simulink library "FasBtc"  (R2022b)
settings: Solver=VariableStepAuto  StartTime=0.0  StopTime=10.0  RelTol=1e-3
undefined symbols (not defined in the file or in its folder): Row
libraries: TuneVar x17, TOP x6, RTC x3, AudioStats x2, FeaturePath x2, HandyTextFile x2, dspmtrx3 x1
settings Model: Creator=kl13806  LastModifiedBy=kl13806
settings SolverCC: AlgebraicLoopSolver=TrustRegion
settings DebuggingCC: UnconnectedInputMsg=warning  UnconnectedOutputMsg=warning  UnconnectedLineMsg=warning  SFMachineParentedDataDiag=warning
settings ModelReferenceCC: EnableRefExpFcnMdlSchedulingChecks=on
settings RTWCC: DLArmComputeVersion=19.05

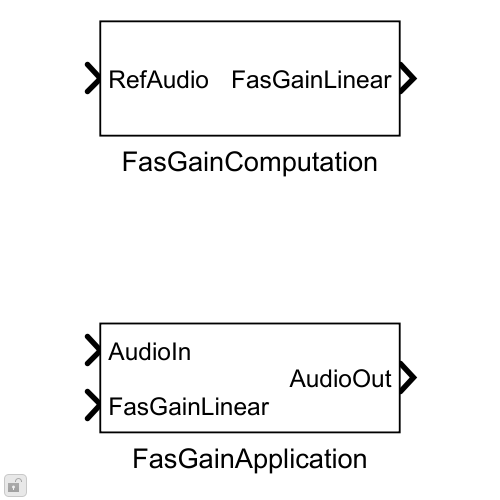
[thumbnail: Simulink's stored preview of the top-level diagram]
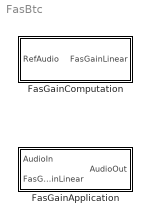
== system FasBtc ==
  FasGainApplication : Subsystem  mask(Blocklib FasGainApplication){Config=[], FeatureName=fas_application_}
      mask prompts: Config "FasGainApplicationConfig"; FeatureName "Feature path name:"
      mask help:
      | The Fresh Air Speaker (FAS) algorithm is designed to limit the output level of selected speaker channels. The level of the remaining channels remains unaffected. This has been implemented in 2 parts - a FAS gain computation block and a FAS gain application block. Refer to the Help section for more information.
      |
      | This limiting is only necessary when windows are open, leading to a reduction in the excursion range of the FAS transducers in order to prevent damage.
      mask init:
      | blkh=gcbh;
      | Config=BTConfig.Assert(blkh,Config);
      | Config.Validate();
      | BTConfig.InitSetFeatureIfPresent(blkh,'FeatureName');
      mask Help:
      | FAS Gain Application:
      | Description:
      | Applies the gain factor to the incoming audio after ramping it using a LPF. Inputs to the block are the gain factor (at framerate) and the input audio. Output from the block is the audio with the gain factors applied.
      | 
      | Mask parameters:
      | 1. FAS enable for each channel (uint32 ; [numChannels x 1]) - Either 0/1 (FAS disable/enable). Will throw an error if number of input audio channels does not match this array size.
      | 2. System parameters like frame size and sample rate are extracted from the input audio.
      | 3. Configuration: The default configuration is defined in FASApplicationConfig.m (FAS computation has a separate configuration file). Please check the file for more details on how to modify the default values.
      | 
      | Tuning support:
      | 1. LPF cut-off frequency - (Hz ; single) Ramps the gain factor
      | 2. FAS enable for each channel - (uint32) Promoted as a mask parameter
      mask Callback Config: BTConfig.CallbackHideIfPresent(gcbh,{'FeatureName'});
      mask TypeOptions FeatureName: FeaturePath/FeatureName
  FasGainComputation : Subsystem  mask(Blocklib FasGainComputation){Config=[], FeatureName=fas_computation_}
      mask prompts: Config "FasGainComputationConfig"; FeatureName "Feature path name:"
      mask help:
      | The Fresh Air Speaker (FAS) algorithm is designed to limit the output level of selected speaker channels. The output level of the remaining channels remains unaffected. This has been implemented in 2 parts - a FAS gain computation block and a FAS gain application block. The audio input to this block is only used to get audio stats (which will define the samplerate of this block).
      |
      | This limiting is only necessary when windows are open, leading to a reduction in the excursion range of the FAS transducers in order to prevent damage.
      mask init:
      | blkh=gcbh;
      | Config=BTConfig.Assert(blkh,Config);
      | Config.Validate();
      | BTConfig.InitSetFeatureIfPresent(blkh,'FeatureName');
      mask Help:
      | FAS Gain computation:
      | Description:
      | Computes the gain factor (based on speed and window status) to be applied to the channels which need pressure protection. Speed input is to be provided (either from the AudioPilot block or from a standalone RTC). The output gain factor is a value between [0,1]. System parameters like frame size and sample rate need to be provided through the mask.
      | 
      | Mask parameters:
      | 1. Configuration: The default configuration is defined in FASComputationConfig.m (FASApplication has a separate configuration file). Please check the file for more details on how to modify the default configuration.
      | 
      | Control support :
      | 1. Window Open status - (uint32) Can be 0 (window not open, FAS not needed) or 1 (window open, FAS needed).
      | 2. Speed In - (single) Current speed of the vehicle
      | 
      | Tuning support:
      | 1. Log minimum value - (single) To ensure that the computed gain in dB does not go to zero
      | 2. Slew Attack - (dB/second) Controls how fast the gain factor increases. TOP is specified in dB/samples.
      | 3. Slew Decay - (dB/second) Controls how fast the gain factor decreases. TOP is specified in dB/samples.
      | 4. Slew Threshold - (dB) If the change in slew is within this threshold, there is no update.
      | 5. Slow slew- (dB/second) Can be ignored for FAS.
      | 6. Speed Threshold (speed units) - Speed beyond which a negative gain is applied
      | 7. Speed Slope - Slope which the speed curve follows for the gain reduction.
      mask Callback Config: BTConfig.CallbackHideIfPresent(gcbh,{'FeatureName'});
      mask TypeOptions FeatureName: FeaturePath/FeatureName

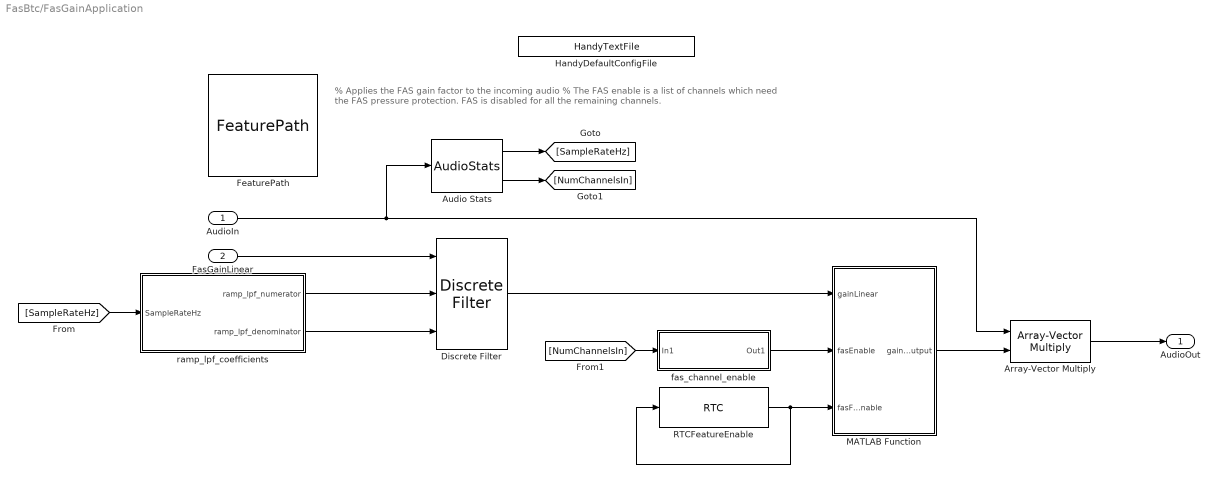
== system FasBtc/FasGainApplication ==
  note: % Applies the FAS gain factor to the incoming audio
      | % The FAS enable is a list of channels which need the FAS pressure protection. FAS is disabled for all the remaining channels.
  AudioIn : Inport
  FasGainLinear : Inport  Port=2  OutDataTypeStr=single
  Array-Vector Multiply : dspmtrx3/Array-Vector Multiply  mode=Mute  saveAsFlag=0  Dimension=2  V_Source=Input port  V_VectFromMask=[0.5 0.25]  roundingMode=Floor  overflowMode=off  firstCoeffSignedness=Auto  firstCoeffDataTypeStr=Inherit: Same word length as input  firstCoeffMin=[]  firstCoeffMax=[]  firstCoeffLastDataTypeStr=Inherit: Same word length as input  prodOutputSignedness=Auto  accumSignedness=Auto  outputSignedness=Auto  outputDataTypeStr=Inherit: Same as product output  outputMin=[]  outputMax=[]  outputLastDataTypeStr=Inherit: Same as product output
  Audio Stats : AudioStats/AudioStats  DoSampleRate=on  TypeSampleRate=Inherit: auto  DoCallRate=off  TypeCallRate=Inherit: auto  DoFrameSize=off  TypeFrameSize=Inherit: auto  DoChannelCount=on  TypeChannelCount=Inherit: auto  DoTaskRateFactor=off  TypeTaskRateFactor=Inherit: auto  MacroNameRoot=AUDIO  MacroNameRootEval='AUDIO'  IsMacroNameEval=off  MacroSampleRate=off  MacroCallRate=off  MacroFrameSize=off  MacroChannelCount=off  MacroTaskRateFactor=off  MacroTaskId=off  ValidateSampleRate=off  ValueSampleRate=[]  ValidateCallRate=off  ValueCallRate=[]  ValidateFrameSize=off  ValueFrameSize=[]  ValidateChannelCount=off  ValueChannelCount=[]  ValidateTaskRateFactor=off  ValueTaskRateFactor=[]
      settings: SourceProductName=Bose Talaria
  Discrete Filter : DiscreteFilter  NumeratorSource=Input port  DenominatorSource=Input port  InputProcessing=Columns as channels (frame based)  FilterStructure=Direct form II transposed  a0EqualsOne=on
      settings: InputPortMap=u0,p1,p3
  FeaturePath : FeaturePath/FeaturePath  FeatureName=fas_application_  IsGroup=off  GroupNumber=-1  IsModule=off  TriggerInit=[-160 -46 -45 61]
      settings: SourceProductName=Bose Talaria
  HandyDefaultConfigFile : HandyTextFile/HandyTextFile  TemplateSource=Config  FileSuffix=Init  OpenDialogOnLoad=off  UseThisBlockName=off  AddGrandParentNamePrefix=off  TheDefaultText=|  ShowInLibBrowser=on
      | % $(FILENAME) Setup model parameters for each "Init" callback (e.g. update diagram)
      | sample_rate_in_hertz = 44100;
      | frame_size = 32;
      | sysin_channel_count = 2;
      settings: SourceProductName=Bose Talaria
  MATLAB Function : MATLAB Function  TreatAsAtomicUnit=on
  RTCFeatureEnable : RTC/RTC  REQ_Priority=RTC_Mask.NormalPriority  RequestAtInit=off  EnableRequest=off  REQElemName1=enable  REQElemType1=uint32  REQElemWidth1=1  REQElemInitial1=1  REQElemType2=uint32  REQElemWidth2=1  REQElemInitial2=[]  REQElemType3=uint32  REQElemWidth3=1  REQElemInitial3=[]  REQElemType4=uint32  REQElemWidth4=1  REQElemInitial4=[]  REQElemType5=uint32  REQElemWidth5=1  REQElemInitial5=[]  REQElemType6=uint32  REQElemWidth6=1  REQElemInitial6=[]  REQElemType7=uint32  REQElemWidth7=1  REQElemInitial7=[]  REQElemType8=uint32  REQElemWidth8=1  REQElemInitial8=[]  REQElemType9=uint32  REQElemWidth9=1  REQElemInitial9=[]  REQElemType10=uint32  REQElemWidth10=1  REQElemInitial10=[]  EnableResponse=on  EnableRSP_StatusIn=off  RSPElemName1=enable  RSPElemType1=uint32  RSPElemWidth1=1  RSPElemType2=uint32  RSPElemWidth2=1  RSPElemType3=uint32  RSPElemWidth3=1  RSPElemType4=uint32  RSPElemWidth4=1  RSPElemType5=uint32  RSPElemWidth5=1  RSPElemType6=uint32  RSPElemWidth6=1  RSPElemType7=uint32  RSPElemWidth7=1  RSPElemType8=uint32  RSPElemWidth8=1  RSPElemType9=uint32  RSPElemWidth9=1  RSPElemType10=uint32  RSPElemWidth10=1  EnableNotification=off  EnableNTF_PrepTrig=off  NTFElemType1=uint32  NTFElemWidth1=1  NTFElemType2=uint32  NTFElemWidth2=1  NTFElemType3=uint32  NTFElemWidth3=1  NTFElemType4=uint32  NTFElemWidth4=1  NTFElemType5=uint32  NTFElemWidth5=1  NTFElemType6=uint32  NTFElemWidth6=1  NTFElemType7=uint32  NTFElemWidth7=1  NTFElemType8=uint32  NTFElemWidth8=1  NTFElemType9=uint32  NTFElemWidth9=1  NTFElemType10=uint32  NTFElemWidth10=1  MaskMessageName=featureEnable
      settings: SourceProductName=Bose Talaria
  fas_channel_enable : Subsystem
  ramp_lpf_coefficients : Subsystem
  AudioOut : Outport
  wires:
  MATLAB Function/1(gainOutput) -> Array-Vector Multiply/2
  Array-Vector Multiply/1 -> AudioOut/1
  Discrete Filter/1 -> MATLAB Function/1(gainLinear)
  fas_channel_enable/1(Out1) -> MATLAB Function/2(fasEnable)
  AudioIn/1 -> Audio Stats/1, Array-Vector Multiply/1
  FasGainLinear/1 -> Discrete Filter/1
  ramp_lpf_coefficients/2(ramp_lpf_denominator) -> Discrete Filter/3
  ramp_lpf_coefficients/1(ramp_lpf_numerator) -> Discrete Filter/2
  Audio Stats/1 -> [SampleRateHz]
  [SampleRateHz] -> ramp_lpf_coefficients/1(SampleRateHz)
  RTCFeatureEnable/1 -> RTCFeatureEnable/1, MATLAB Function/3(fasFeatureEnable)
  Audio Stats/2 -> [NumChannelsIn]
  [NumChannelsIn] -> fas_channel_enable/1(In1)

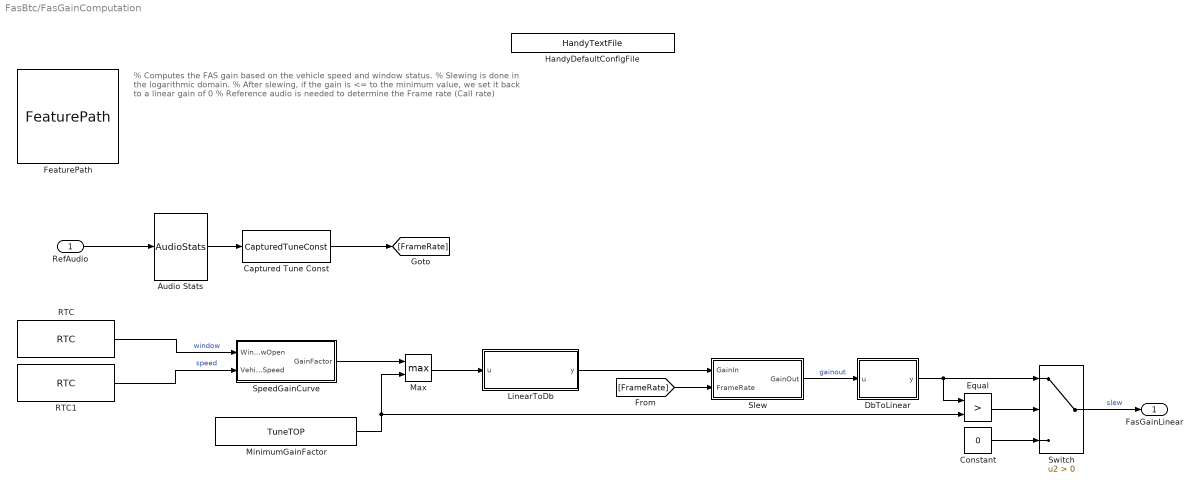
== system FasBtc/FasGainComputation ==
  note: % Computes the FAS gain based on the vehicle speed and window status.
      | % Slewing is done in the logarithmic domain.
      | % After slewing, if the gain is <= to the minimum value, we set it back to a linear gain of 0
      | % Reference audio is needed to determine the Frame rate (Call rate)
  RefAudio : Inport
  Audio Stats : AudioStats/AudioStats  DoSampleRate=off  TypeSampleRate=Inherit: auto  DoCallRate=on  TypeCallRate=Inherit: auto  DoFrameSize=off  TypeFrameSize=Inherit: auto  DoChannelCount=off  TypeChannelCount=Inherit: auto  DoTaskRateFactor=off  TypeTaskRateFactor=Inherit: auto  MacroNameRoot=AUDIO  MacroNameRootEval='AUDIO'  IsMacroNameEval=off  MacroSampleRate=off  MacroCallRate=off  MacroFrameSize=off  MacroChannelCount=off  MacroTaskRateFactor=off  MacroTaskId=off  ValidateSampleRate=off  ValueSampleRate=[]  ValidateCallRate=off  ValueCallRate=[]  ValidateFrameSize=off  ValueFrameSize=[]  ValidateChannelCount=off  ValueChannelCount=[]  ValidateTaskRateFactor=off  ValueTaskRateFactor=[]
      settings: SourceProductName=Bose Talaria
  Captured Tune Const : TuneVar/CapturedTuneConst  TriggerInit=[-125 -48 -25 -12]  Role=Automatic
      settings: SourceProductName=Bose Talaria
  Constant : Constant  Value=0  OutDataTypeStr=single
  DbToLinear : MATLAB Function  TreatAsAtomicUnit=on
  Equal : RelationalOperator  Operator=>  OutDataTypeStr=boolean  RndMeth=Simplest  InputSameDT=off
  FeaturePath : FeaturePath/FeaturePath  FeatureName=fas_computation_  IsGroup=off  GroupNumber=-1  IsModule=off  TriggerInit=[-380 -231 -265 -124]
      settings: SourceProductName=Bose Talaria
  HandyDefaultConfigFile : HandyTextFile/HandyTextFile  TemplateSource=Config  FileSuffix=Init  OpenDialogOnLoad=off  UseThisBlockName=off  AddGrandParentNamePrefix=off  TheDefaultText=|  ShowInLibBrowser=on
      | % $(FILENAME) Setup model parameters for each "Init" callback (e.g. update diagram)
      | sample_rate_in_hertz = 44100;
      | frame_size = 32;
      | sysin_channel_count = 2;
      settings: SourceProductName=Bose Talaria
  LinearToDb : MATLAB Function  TreatAsAtomicUnit=on
  Max : MinMax  Function=max  Inputs=2
  MinimumGainFactor : TuneVar/TuneTOP  TriggerInit=[-155 164 5 196]  TopName=min_gain_factor  TuneName=min_gain_factor  DataType=single  TunabilityNumber=1  MinValue=[]  MaxValue=[]  BankNumber=0  PreOverlay=false  PostOverlay=false  UseSameName=on  MaskValue=Config.DefaultGainMinValue
      settings: SourceProductName=Bose Talaria
  RTC : RTC/RTC  REQ_Priority=RTC_Mask.NormalPriority  RequestAtInit=off  EnableRequest=off  REQElemName1=windowOpen  REQElemType1=uint32  REQElemWidth1=1  REQElemInitial1=[]  REQElemType2=uint32  REQElemWidth2=1  REQElemInitial2=[]  REQElemType3=uint32  REQElemWidth3=1  REQElemInitial3=[]  REQElemType4=uint32  REQElemWidth4=1  REQElemInitial4=[]  REQElemType5=uint32  REQElemWidth5=1  REQElemInitial5=[]  REQElemType6=uint32  REQElemWidth6=1  REQElemInitial6=[]  REQElemType7=uint32  REQElemWidth7=1  REQElemInitial7=[]  REQElemType8=uint32  REQElemWidth8=1  REQElemInitial8=[]  REQElemType9=uint32  REQElemWidth9=1  REQElemInitial9=[]  REQElemType10=uint32  REQElemWidth10=1  REQElemInitial10=[]  EnableResponse=off  EnableRSP_StatusIn=off  RSPElemName1=windowStatus  RSPElemType1=uint32  RSPElemWidth1=1  RSPElemType2=uint32  RSPElemWidth2=1  RSPElemType3=uint32  RSPElemWidth3=1  RSPElemType4=uint32  RSPElemWidth4=1  RSPElemType5=uint32  RSPElemWidth5=1  RSPElemType6=uint32  RSPElemWidth6=1  RSPElemType7=uint32  RSPElemWidth7=1  RSPElemType8=uint32  RSPElemWidth8=1  RSPElemType9=uint32  RSPElemWidth9=1  RSPElemType10=uint32  RSPElemWidth10=1  EnableNotification=off  EnableNTF_PrepTrig=off  NTFElemType1=uint32  NTFElemWidth1=1  NTFElemType2=uint32  NTFElemWidth2=1  NTFElemType3=uint32  NTFElemWidth3=1  NTFElemType4=uint32  NTFElemWidth4=1  NTFElemType5=uint32  NTFElemWidth5=1  NTFElemType6=uint32  NTFElemWidth6=1  NTFElemType7=uint32  NTFElemWidth7=1  NTFElemType8=uint32  NTFElemWidth8=1  NTFElemType9=uint32  NTFElemWidth9=1  NTFElemType10=uint32  NTFElemWidth10=1  MaskMessageName=WindowOpen
      settings: SourceProductName=Bose Talaria
  RTC1 : RTC/RTC  REQ_Priority=RTC_Mask.NormalPriority  RequestAtInit=off  EnableRequest=off  REQElemName1=speedIn  REQElemType1=single  REQElemWidth1=1  REQElemInitial1=0  REQElemType2=single  REQElemWidth2=1  REQElemInitial2=[]  REQElemType3=uint32  REQElemWidth3=1  REQElemInitial3=[]  REQElemType4=uint32  REQElemWidth4=1  REQElemInitial4=[]  REQElemType5=uint32  REQElemWidth5=1  REQElemInitial5=[]  REQElemType6=uint32  REQElemWidth6=1  REQElemInitial6=[]  REQElemType7=uint32  REQElemWidth7=1  REQElemInitial7=[]  REQElemType8=uint32  REQElemWidth8=1  REQElemInitial8=[]  REQElemType9=uint32  REQElemWidth9=1  REQElemInitial9=[]  REQElemType10=uint32  REQElemWidth10=1  REQElemInitial10=[]  EnableResponse=off  EnableRSP_StatusIn=off  RSPElemName1=FANLevel  RSPElemType1=single  RSPElemWidth1=1  RSPElemType2=uint32  RSPElemWidth2=1  RSPElemType3=uint32  RSPElemWidth3=1  RSPElemType4=uint32  RSPElemWidth4=1  RSPElemType5=uint32  RSPElemWidth5=1  RSPElemType6=uint32  RSPElemWidth6=1  RSPElemType7=uint32  RSPElemWidth7=1  RSPElemType8=uint32  RSPElemWidth8=1  RSPElemType9=uint32  RSPElemWidth9=1  RSPElemType10=uint32  RSPElemWidth10=1  EnableNotification=off  EnableNTF_PrepTrig=off  NTFElemType1=uint32  NTFElemWidth1=1  NTFElemType2=uint32  NTFElemWidth2=1  NTFElemType3=uint32  NTFElemWidth3=1  NTFElemType4=uint32  NTFElemWidth4=1  NTFElemType5=uint32  NTFElemWidth5=1  NTFElemType6=uint32  NTFElemWidth6=1  NTFElemType7=uint32  NTFElemWidth7=1  NTFElemType8=uint32  NTFElemWidth8=1  NTFElemType9=uint32  NTFElemWidth9=1  NTFElemType10=uint32  NTFElemWidth10=1  MaskMessageName=SetSpeedIn
      settings: SourceProductName=Bose Talaria
  Slew : Subsystem
  SpeedGainCurve : Subsystem
  Switch : Switch  Criteria=u2 > Threshold  SaturateOnIntegerOverflow=off  InputSameDT=off
  FasGainLinear : Outport
  wires:
  [FrameRate] -> Slew/2(FrameRate)
  Audio Stats/1 -> Captured Tune Const/1
  RefAudio/1 -> Audio Stats/1
  Captured Tune Const/1 -> [FrameRate]
  DbToLinear/1(y) -> Equal/1, Switch/1
  Max/1 -> LinearToDb/1(u)
  Constant/1 -> Switch/3
  Equal/1 -> Switch/2
  Slew/1(GainOut) -> DbToLinear/1(u)  "gainout"
  LinearToDb/1(y) -> Slew/1(GainIn)
  MinimumGainFactor/1 -> Equal/2, Max/2
  Switch/1 -> FasGainLinear/1  "slew"
  SpeedGainCurve/1(GainFactor) -> Max/1
  RTC1/1 -> SpeedGainCurve/2(VehicleSpeed)  "speed"
  RTC/1 -> SpeedGainCurve/1(WindowOpen)  "window"

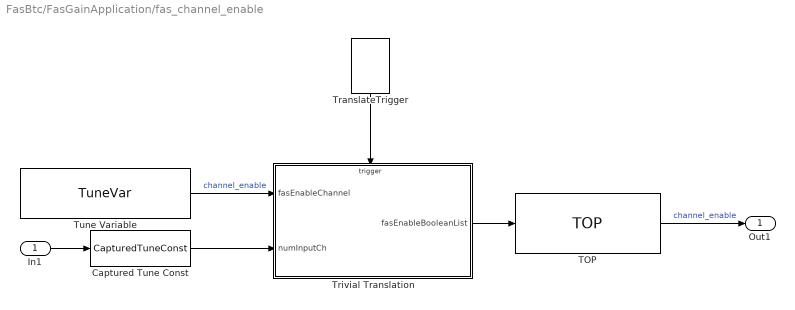
== system FasBtc/FasGainApplication/fas_channel_enable ==
  In1 : Inport
  Captured Tune Const : TuneVar/CapturedTuneConst  TriggerInit=[45 92 145 128]  Role=Automatic
      settings: SourceProductName=Bose Talaria
  TOP : TOP/TOP  TriggerInit=[470 55 615 115]  TopName=channel_enable  DataType=uint32  BankNumber=0  PreOverlay=false  PostOverlay=false  Role=Automatic
      settings: SourceProductName=Bose Talaria
  TranslateTrigger : TuneVar/TranslateTrigger  TriggerInit=[306 -100 344 -45]
      settings: SourceProductName=Bose Talaria
  Trivial Translation : MATLAB Function  TreatAsAtomicUnit=on
  Tune Variable : TuneVar/TuneVar  TuneName=channel_enable  SpecifyMaxSize=off  VariableDim=1 (Row)  MaxSize=[1 1]  TunabilityNumber=1  MinValue=[]  MaxValue=[]  TriggerInit=[-25 30 145 80]  MaskValue=Config.DefautFasEnable
      settings: SourceProductName=Bose Talaria
  Out1 : Outport  VectorParamsAs1DForOutWhenUnconnected=off
  wires:
  TranslateTrigger/1 -> Trivial Translation/Trigger
  Trivial Translation/1(fasEnableBooleanList) -> TOP/1
  Tune Variable/1 -> Trivial Translation/1(fasEnableChannel)  "channel_enable"
  TOP/1 -> Out1/1  "channel_enable"
  In1/1 -> Captured Tune Const/1
  Captured Tune Const/1 -> Trivial Translation/2(numInputCh)

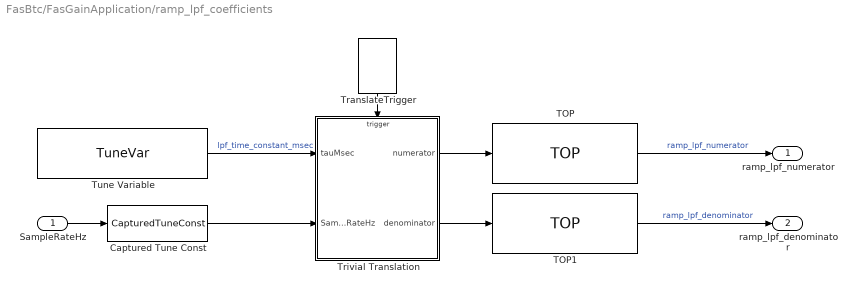
== system FasBtc/FasGainApplication/ramp_lpf_coefficients ==
  SampleRateHz : Inport
  Captured Tune Const : TuneVar/CapturedTuneConst  TriggerInit=[55 72 155 108]  Role=Automatic
      settings: SourceProductName=Bose Talaria
  TOP : TOP/TOP  TriggerInit=[440 -10 585 50]  TopName=ramp_lpf_numerator  DataType=single  BankNumber=0  PreOverlay=false  PostOverlay=false  Role=Automatic
      settings: SourceProductName=Bose Talaria
  TOP1 : TOP/TOP  TriggerInit=[440 60 585 120]  TopName=ramp_lpf_denominator  DataType=single  BankNumber=0  PreOverlay=false  PostOverlay=false  Role=Automatic
      settings: SourceProductName=Bose Talaria
  TranslateTrigger : TuneVar/TranslateTrigger  TriggerInit=[306 -95 344 -40]
      settings: SourceProductName=Bose Talaria
  Trivial Translation : MATLAB Function  TreatAsAtomicUnit=on
  Tune Variable : TuneVar/TuneVar  TuneName=lpf_time_constant_msec  SpecifyMaxSize=off  VariableDim=1 (Row)  MaxSize=[1 1]  TunabilityNumber=1  MinValue=[]  MaxValue=[]  TriggerInit=[-15 -5 155 45]  MaskValue=Config.DefaultLpfTimeConstMsec
      settings: SourceProductName=Bose Talaria
  ramp_lpf_numerator : Outport  VectorParamsAs1DForOutWhenUnconnected=off
  ramp_lpf_denominator : Outport  Port=2
  wires:
  TOP1/1 -> ramp_lpf_denominator/1  "ramp_lpf_denominator"
  Trivial Translation/2(denominator) -> TOP1/1
  TranslateTrigger/1 -> Trivial Translation/Trigger
  Trivial Translation/1(numerator) -> TOP/1
  Tune Variable/1 -> Trivial Translation/1(tauMsec)  "lpf_time_constant_msec"
  TOP/1 -> ramp_lpf_numerator/1  "ramp_lpf_numerator"
  SampleRateHz/1 -> Captured Tune Const/1
  Captured Tune Const/1 -> Trivial Translation/2(SampleRateHz)

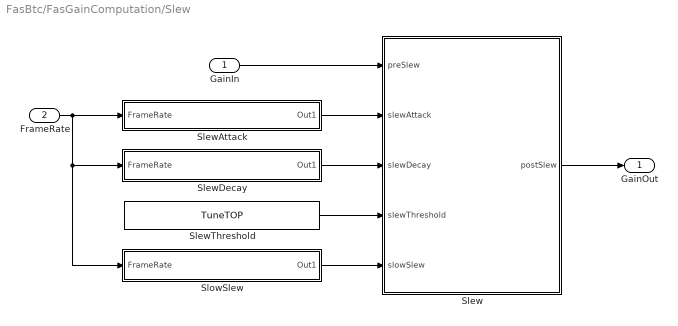
== system FasBtc/FasGainComputation/Slew ==
  GainIn : Inport
  FrameRate : Inport  Port=2
  Slew : MATLAB Function  TreatAsAtomicUnit=on
  SlewAttack : Subsystem
  SlewDecay : Subsystem
  SlewThreshold : TuneVar/TuneTOP  TriggerInit=[-130 251 65 279]  TopName=slew_threshold_db  TuneName=slew_threshold_db  DataType=single  TunabilityNumber=1  MinValue=[]  MaxValue=[]  BankNumber=0  PreOverlay=false  PostOverlay=false  UseSameName=on  MaskValue=Config.DefaultSlewThreshold
      settings: SourceProductName=Bose Talaria
  SlowSlew : Subsystem
  GainOut : Outport
  wires:
  SlowSlew/1(Out1) -> Slew/5(slowSlew)
  SlewThreshold/1 -> Slew/4(slewThreshold)
  SlewDecay/1(Out1) -> Slew/3(slewDecay)
  SlewAttack/1(Out1) -> Slew/2(slewAttack)
  Slew/1(postSlew) -> GainOut/1
  GainIn/1 -> Slew/1(preSlew)
  FrameRate/1 -> SlewAttack/1(FrameRate), SlewDecay/1(FrameRate), SlowSlew/1(FrameRate)

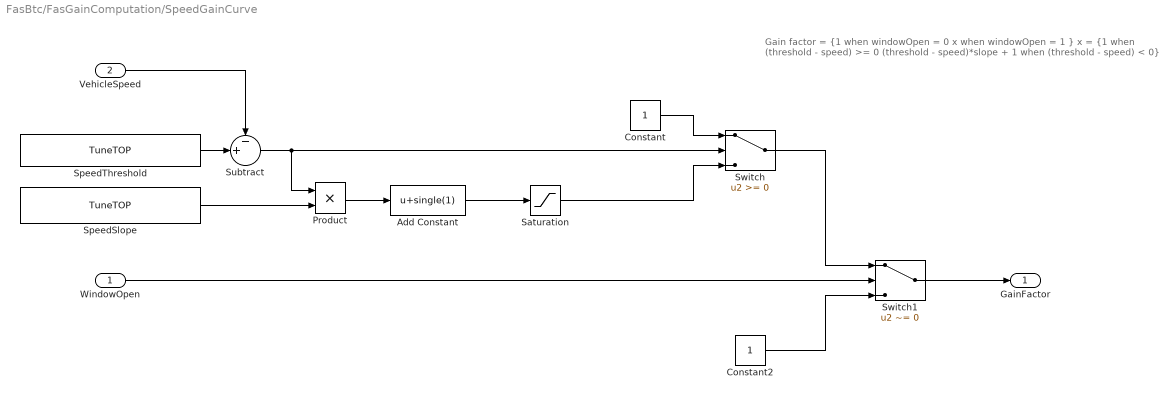
== system FasBtc/FasGainComputation/SpeedGainCurve ==
  note: Gain factor = {1 			when windowOpen = 0
      |                        x		 	when windowOpen = 1 }
      | x		    = {1								when (threshold - speed) >= 0
      | 			 (threshold - speed)*slope + 1		when (threshold - speed) < 0}
  WindowOpen : Inport
  VehicleSpeed : Inport  Port=2
  Add Constant : Bias  Bias=single(1)  SaturateOnIntegerOverflow=off
  Constant : Constant  OutDataTypeStr=single
  Constant2 : Constant  OutDataTypeStr=single
  Product : Product
  Saturation : Saturate  UpperLimit=1  LowerLimit=0  OutDataTypeStr=single
  SpeedSlope : TuneVar/TuneTOP  TriggerInit=[-150 57 30 93]  TopName=speed_slope  TuneName=speed_slope  DataType=single  TunabilityNumber=1  MinValue=[]  MaxValue=[]  BankNumber=0  PreOverlay=false  PostOverlay=false  UseSameName=on  MaskValue=Config.DefaultSpeedGainThreshold
      settings: SourceProductName=Bose Talaria
  SpeedThreshold : TuneVar/TuneTOP  TriggerInit=[-150 4 30 36]  TopName=speed_threshold  TuneName=speed_threshold  DataType=single  TunabilityNumber=1  MinValue=[]  MaxValue=[]  BankNumber=0  PreOverlay=false  PostOverlay=false  UseSameName=on  MaskValue=Config.DefaultSpeedGainThreshold
      settings: SourceProductName=Bose Talaria
  Subtract : Sum  Inputs=-+|
  Switch : Switch  OutDataTypeStr=single  SaturateOnIntegerOverflow=off  InputSameDT=off
  Switch1 : Switch  Criteria=u2 ~= 0  OutDataTypeStr=single  SaturateOnIntegerOverflow=off  InputSameDT=off
  GainFactor : Outport
  wires:
  Saturation/1 -> Switch/3
  Add Constant/1 -> Saturation/1
  Constant2/1 -> Switch1/3
  WindowOpen/1 -> Switch1/2
  Switch/1 -> Switch1/1
  Switch1/1 -> GainFactor/1
  Constant/1 -> Switch/1
  Product/1 -> Add Constant/1
  SpeedSlope/1 -> Product/2
  Subtract/1 -> Product/1, Switch/2
  VehicleSpeed/1 -> Subtract/1
  SpeedThreshold/1 -> Subtract/2

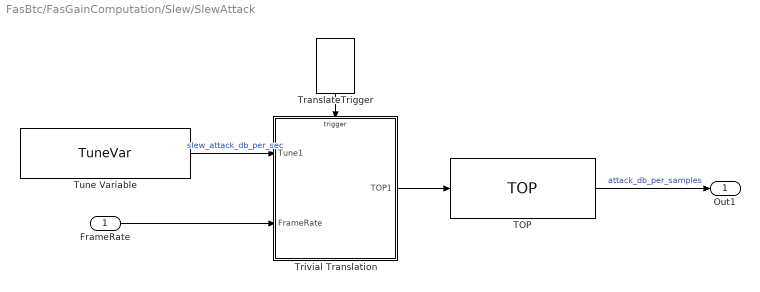
== system FasBtc/FasGainComputation/Slew/SlewAttack ==
  FrameRate : Inport
  TOP : TOP/TOP  TriggerInit=[440 20 585 80]  TopName=attack_db_per_samples  DataType=single  BankNumber=0  PreOverlay=false  PostOverlay=false  Role=Automatic
      settings: SourceProductName=Bose Talaria
  TranslateTrigger : TuneVar/TranslateTrigger  TriggerInit=[306 -100 344 -45]
      settings: SourceProductName=Bose Talaria
  Trivial Translation : MATLAB Function  TreatAsAtomicUnit=on
  Tune Variable : TuneVar/TuneVar  TuneName=slew_attack_db_per_sec  SpecifyMaxSize=off  VariableDim=1 (Row)  MaxSize=[1 1]  TunabilityNumber=1  MinValue=[]  MaxValue=[]  TriggerInit=[10 -10 180 40]  MaskValue=Config.DefaultSlewAttackDbPerSec
      settings: SourceProductName=Bose Talaria
  Out1 : Outport  VectorParamsAs1DForOutWhenUnconnected=off
  wires:
  TranslateTrigger/1 -> Trivial Translation/Trigger
  Trivial Translation/1(TOP1) -> TOP/1
  Tune Variable/1 -> Trivial Translation/1(Tune1)  "slew_attack_db_per_sec"
  TOP/1 -> Out1/1  "attack_db_per_samples"
  FrameRate/1 -> Trivial Translation/2(FrameRate)

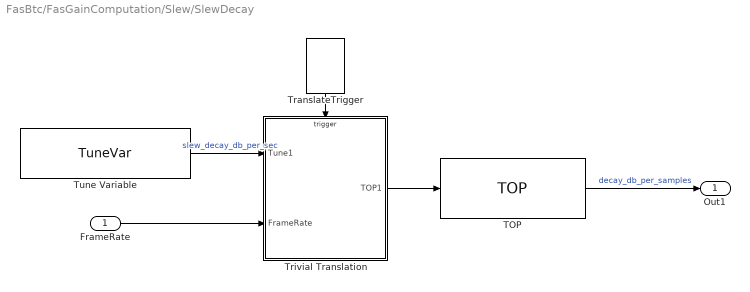
== system FasBtc/FasGainComputation/Slew/SlewDecay ==
  FrameRate : Inport
  TOP : TOP/TOP  TriggerInit=[440 20 585 80]  TopName=decay_db_per_samples  DataType=single  BankNumber=0  PreOverlay=false  PostOverlay=false  Role=Automatic
      settings: SourceProductName=Bose Talaria
  TranslateTrigger : TuneVar/TranslateTrigger  TriggerInit=[306 -100 344 -45]
      settings: SourceProductName=Bose Talaria
  Trivial Translation : MATLAB Function  TreatAsAtomicUnit=on
  Tune Variable : TuneVar/TuneVar  TuneName=slew_decay_db_per_sec  SpecifyMaxSize=off  VariableDim=1 (Row)  MaxSize=[1 1]  TunabilityNumber=1  MinValue=[]  MaxValue=[]  TriggerInit=[20 -10 190 40]  MaskValue=Config.DefaulySlewDecayDbPerSec
      settings: SourceProductName=Bose Talaria
  Out1 : Outport  VectorParamsAs1DForOutWhenUnconnected=off
  wires:
  TranslateTrigger/1 -> Trivial Translation/Trigger
  Trivial Translation/1(TOP1) -> TOP/1
  Tune Variable/1 -> Trivial Translation/1(Tune1)  "slew_decay_db_per_sec"
  TOP/1 -> Out1/1  "decay_db_per_samples"
  FrameRate/1 -> Trivial Translation/2(FrameRate)

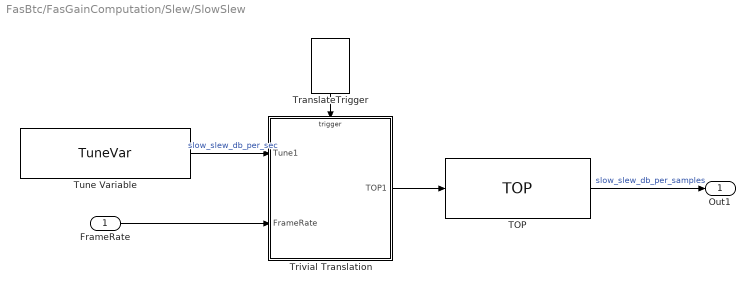
== system FasBtc/FasGainComputation/Slew/SlowSlew ==
  FrameRate : Inport
  TOP : TOP/TOP  TriggerInit=[440 20 585 80]  TopName=slow_slew_db_per_samples  DataType=single  BankNumber=0  PreOverlay=false  PostOverlay=false  Role=Automatic
      settings: SourceProductName=Bose Talaria
  TranslateTrigger : TuneVar/TranslateTrigger  TriggerInit=[306 -100 344 -45]
      settings: SourceProductName=Bose Talaria
  Trivial Translation : MATLAB Function  TreatAsAtomicUnit=on
  Tune Variable : TuneVar/TuneVar  TuneName=slow_slew_db_per_sec  SpecifyMaxSize=off  VariableDim=1 (Row)  MaxSize=[1 1]  TunabilityNumber=1  MinValue=[]  MaxValue=[]  TriggerInit=[15 -10 185 40]  MaskValue=Config.DefaultSlewSlowDbPerSec
      settings: SourceProductName=Bose Talaria
  Out1 : Outport  VectorParamsAs1DForOutWhenUnconnected=off
  wires:
  TranslateTrigger/1 -> Trivial Translation/Trigger
  Trivial Translation/1(TOP1) -> TOP/1
  Tune Variable/1 -> Trivial Translation/1(Tune1)  "slow_slew_db_per_sec"
  TOP/1 -> Out1/1  "slow_slew_db_per_samples"
  FrameRate/1 -> Trivial Translation/2(FrameRate)

== matlab function FasBtc/FasGainComputation/DbToLinear ==
  data: u input; y output
function y = dB_to_linear(u)

% Convert gain from dB to linear
y = single( 10 ^ (u/20) );

== matlab function FasBtc/FasGainComputation/LinearToDb ==
  data: u input; y output
function y = linear_to_dB(u)

% Convert gain from linear to dB
y = single(20 * log10(u));

== matlab function FasBtc/FasGainApplication/MATLAB Function ==
  data: gainLinear input; fasEnable input; gainOutput output; fasFeatureEnable input
function gainOutput = fcn(gainLinear, fasEnable, fasFeatureEnable)
% For channels which have FAS enabled, use the FAS gain. For channels which
% have FAS disabled, use a default gain of 1.
% gainOutput size is also defined in the Edit Data options.

gainOutput = coder.nullcopy(zeros(size(fasEnable),'single'));
gainOutput = ones(size(fasEnable),'single');
if fasFeatureEnable == uint32(1)
    channelsWithFas = fasEnable == 1;
    gainOutput(channelsWithFas) = (gainLinear);
end

== matlab function FasBtc/FasGainApplication/fas_channel_enable/Trivial Translation ==
  data: fasEnableBooleanList output; fasEnableChannel input; numInputCh input
  events: trigger input FUNCTION_CALL_EVENT
function fasEnableBooleanList  = fcn(fasEnableChannel, numInputCh)
%#codegen
% "fasEnableChannel" : integer array containing a '1' or a '0' based on
% whether FAS is needed or not

argName = 'FAS';

% Ensure each channel is present in the enable list
numChannelEnables = numel(fasEnableChannel.Value);
if (numChannelEnables ~= numInputCh)
   TranslateError(['Error in %s : Number of channels in the channel map [%d] does'... 
       'not match number of input channels [%d]. Make sure all channels '...
       'are present in the channel-map array.'], argName, numChannelEnables, numInputCh);
end

fasEnableBooleanList = fasEnableChannel.Value;

== matlab function FasBtc/FasGainComputation/Slew/SlewAttack/Trivial Translation ==
  data: TOP1 output; Tune1 input; FrameRate input
  events: trigger input FUNCTION_CALL_EVENT
function TOP1  = fcn(Tune1, FrameRate)

% Translation to convert from attack_db_per_second to attack_db_per_sample
TOP1 = Tune1.Value / FrameRate;

== matlab function FasBtc/FasGainComputation/Slew/SlewDecay/Trivial Translation ==
  data: TOP1 output; Tune1 input; FrameRate input
  events: trigger input FUNCTION_CALL_EVENT
function TOP1  = fcn(Tune1, FrameRate)

% Translation to convert from slew_decay_db_per_second to 
% slew_decay_db_per_sample
TOP1 = -abs(Tune1.Value / FrameRate);

== matlab function FasBtc/FasGainComputation/Slew/SlowSlew/Trivial Translation ==
  data: TOP1 output; Tune1 input; FrameRate input
  events: trigger input FUNCTION_CALL_EVENT
function TOP1  = fcn(Tune1, FrameRate)

% Translation to convert from slow_slew_db_per_second to 
% slow_slew_db_per_sample
TOP1 = (Tune1.Value / FrameRate);

== matlab function FasBtc/FasGainApplication/ramp_lpf_coefficients/Trivial Translation ==
  data: numerator output; tauMsec input; denominator output; SampleRateHz input
  events: trigger input FUNCTION_CALL_EVENT
function [numerator, denominator] = fcn(tauMsec, SampleRateHz)
%#codegen

% Convert lpf time constant into numerator and 
% denominator 
tauSec = tauMsec.Value / 1000;
fcHz = 1 / tauSec;
wc = 2 * pi * fcHz / SampleRateHz;
Coef = (1 - sin(wc)) / cos(wc);

numerator = [(1-Coef)] ;
denominator = [1, -Coef];

== matlab function FasBtc/FasGainComputation/Slew/Slew ==
  data: preSlew input size=1; slewAttack input =slewAttack; slewDecay input =slewDecay; slewThreshold input =slewThreshold; slowSlew input size=1 =slowSlew; postSlew output
function postSlew = Slew(preSlew, ...
	slewAttack, slewDecay, slewThreshold, slowSlew)
	
persistent prevChange prevDelta prevPostSlew;
if isempty(prevChange); prevChange = single(0);  end
if isempty(prevDelta); prevDelta = single(0);  end
if isempty(prevPostSlew); prevPostSlew = single(0);  end

delta = preSlew - prevPostSlew;

if delta > 0                              % setup for positive delta
	change = min(slewAttack, delta);
	slowSlew = min(slowSlew, delta);
else                                      % setup for negative delta
	change = max(slewDecay, delta);
	slowSlew = max(-slowSlew, delta);
end

if prevDelta*delta > 0					  % did we reach our target?
	slew = single(prevChange);                    % no, continue the current path
else                                      % otherwise, we have reached our target
    slew = slowSlew;  
end

if (abs(delta) <= slewThreshold) ...		% are we within the zone?
		&& (abs(slew) < abs(change))          % is change still bigger than slew?
	change = slew;                        % freeze or continue the current
end

prevDelta = delta;
prevChange = change;

prevPostSlew = prevPostSlew + change;
postSlew = prevPostSlew;
end
